simulink model "hw_BuildIn_Gyro"  (R2020b)
settings: Solver=FixedStepAuto  StartTime=0.0  StopTime=inf  RelTol=1e-3  EnableMultiTasking=on
libraries: arduinolib x10, simulink x4
settings Model: SILPILModeSetting=veronly  EnablePacing=on  ExtModeTrigDuration=2  Creator=IDE-Admin  LastModifiedBy=helve
settings OptimizationCC: EnhancedBackFolding=on  PassReuseOutputArgsAs=Individual arguments  ZeroExternalMemoryAtStartup=off  ZeroInternalMemoryAtStartup=off  MaxStackSize=64  OptimizeBlockOrder=speed  DifferentSizesBufferReuse=on  OptimizationCustomize=off  EfficientTunableParamExpr=on
settings DebuggingCC: ParameterTunabilityLossMsg=error
settings HardwareCC: ProdBitPerPointer=32  ProdBitPerSizeT=32  ProdBitPerPtrDiffT=32  ProdLargestAtomicInteger=Long  ProdLargestAtomicFloat=Double  ProdWordSize=32  ProdHWDeviceType=ARM Compatible->ARM Cortex
settings SFSimCC: MATLABDynamicMemAlloc=off
settings RTWCC: Description=Embedded Coder  SystemTargetFile=ert.tlc  HardwareBoard=Arduino Nano 33 IoT  TemplateMakefile=ert_default_tmf  Toolchain=Arduino ARM  BuildConfiguration=Faster Runs
settings CodeAppCC: ForceParamTrailComments=on  IgnoreCustomStorageClasses=off  OperatorAnnotations=on  SimulinkDataObjDesc=on  SFDataObjDesc=on  InsertBlockDesc=on
settings ERTTargetCC: SupportContinuousTime=on  SupportVariableSizeSignals=on  ExtModeTransport=3  ExtModeStaticAllocSize=8192  ExtModeMexFile=ext_xcp  ExtModeIntrfLevel=Level2 - Open

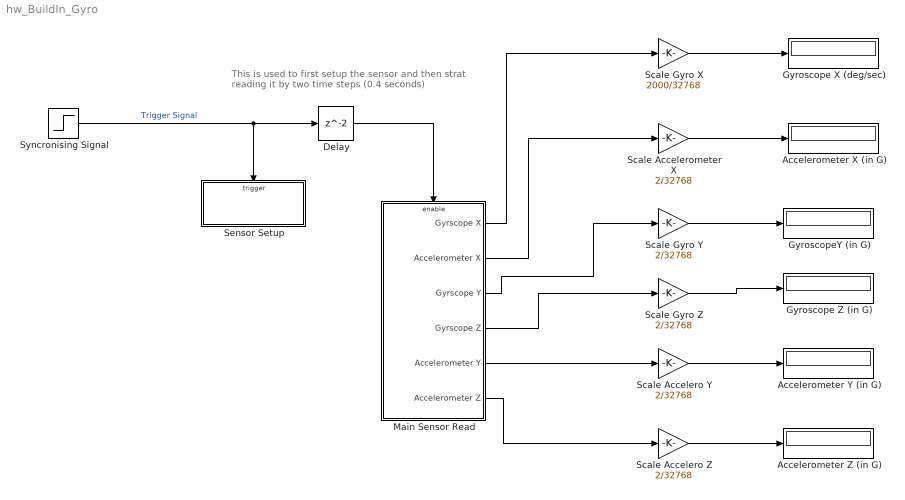
== system hw_BuildIn_Gyro ==
  note: This is used to first setup the sensor and
      | then strat reading it by two time steps (0.4 seconds)
  Accelerometer X (in G) : Display
  Accelerometer Y (in G) : Display
  Accelerometer Z (in G) : Display
  Delay : Delay
  Gyroscope X (deg/sec) : Display
  Gyroscope Z (in G) : Display
  GyroscopeY (in G) : Display
  Main Sensor Read : Subsystem  TreatAsAtomicUnit=on
  Scale Accelero Y : Gain  Gain=2/32768  OutDataTypeStr=single
  Scale Accelero Z : Gain  Gain=2/32768  OutDataTypeStr=single
  Scale Accelerometer X : Gain  Gain=2/32768  OutDataTypeStr=single
  Scale Gyro X : Gain  Gain=2000/32768  OutDataTypeStr=single
  Scale Gyro Y : Gain  Gain=2/32768  OutDataTypeStr=single
  Scale Gyro Z : Gain  Gain=2/32768  OutDataTypeStr=single
  Sensor Setup : Subsystem  TreatAsAtomicUnit=on
  Syncronising Signal : Step
  wires:
  Syncronising Signal/1 -> Sensor Setup/Trigger, Delay/1  "Trigger Signal"
  Delay/1 -> Main Sensor Read/Enable
  Main Sensor Read/1(Gyrscope X) -> Scale Gyro X/1
  Scale Gyro X/1 -> Gyroscope X (deg/sec)/1
  Scale Accelerometer X/1 -> Accelerometer X (in G)/1
  Main Sensor Read/2(Accelerometer X) -> Scale Accelerometer X/1
  Scale Gyro Y/1 -> GyroscopeY (in G)/1
  Main Sensor Read/3(Gyrscope Y) -> Scale Gyro Y/1
  Scale Gyro Z/1 -> Gyroscope Z (in G)/1
  Main Sensor Read/4(Gyrscope Z) -> Scale Gyro Z/1
  Scale Accelero Y/1 -> Accelerometer Y (in G)/1
  Main Sensor Read/5(Accelerometer Y) -> Scale Accelero Y/1
  Scale Accelero Z/1 -> Accelerometer Z (in G)/1
  Main Sensor Read/6(Accelerometer Z) -> Scale Accelero Z/1

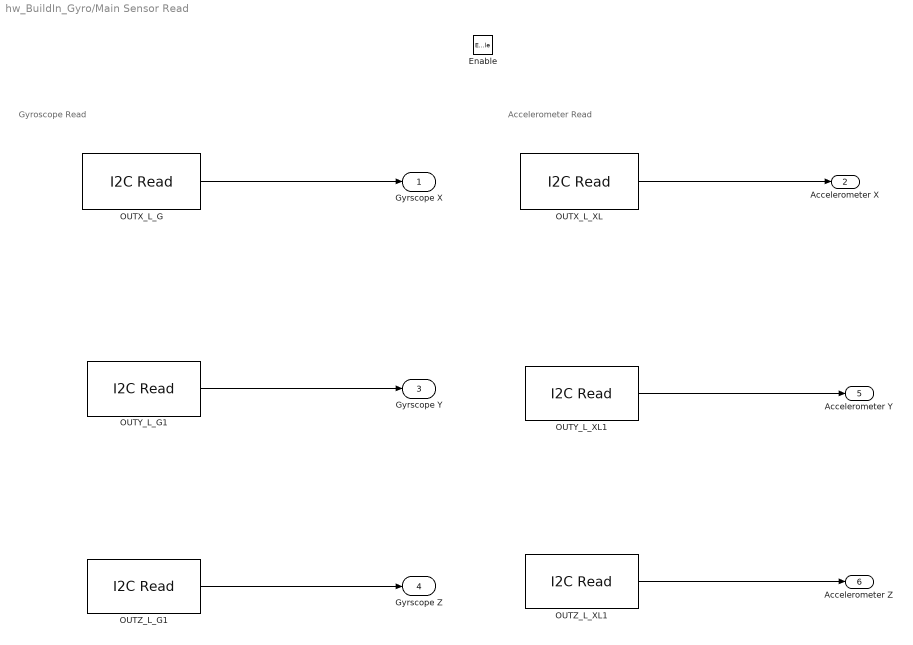
== system hw_BuildIn_Gyro/Main Sensor Read ==
  note: Gyroscope Read
  note: Accelerometer Read
  Enable : EnablePort
  OUTX_L_G : arduinolib/I2C Read  I2CModule=0  Mode=Master  SlaveAddress=0b01101010  SlaveByteOrder=LittleEndian  Direction=Receiver  RegisterAddressMode=on  RegisterAddress=0x22  SlaveDataType=int16  DataLength=1  NoAck=off  RepeatedStart=off  OutputStatus=off  blockPlatform=arduino  SampleTime=-1
      settings: SourceProductBaseCode=ARDUINO
      settings: AttributesFormatString=|
      | %<RegisterAddress>
      | %<SlaveDataType>
  OUTX_L_XL : arduinolib/I2C Read  I2CModule=0  Mode=Master  SlaveAddress=0b01101010  SlaveByteOrder=LittleEndian  Direction=Receiver  RegisterAddressMode=on  RegisterAddress=0x28  SlaveDataType=int16  DataLength=1  NoAck=off  RepeatedStart=off  OutputStatus=off  blockPlatform=arduino  SampleTime=-1
      settings: SourceProductBaseCode=ARDUINO
      settings: AttributesFormatString=|
      | %<RegisterAddress>
      | %<SlaveDataType>
  OUTY_L_G1 : arduinolib/I2C Read  I2CModule=0  Mode=Master  SlaveAddress=0b01101010  SlaveByteOrder=LittleEndian  Direction=Receiver  RegisterAddressMode=on  RegisterAddress=0x24  SlaveDataType=int16  DataLength=1  NoAck=off  RepeatedStart=off  OutputStatus=off  blockPlatform=ARDUINO  SampleTime=-1
      settings: SourceProductBaseCode=ARDUINO
      settings: AttributesFormatString=|
      | %<RegisterAddress>
      | %<SlaveDataType>
  OUTY_L_XL1 : arduinolib/I2C Read  I2CModule=0  Mode=Master  SlaveAddress=0b01101010  SlaveByteOrder=LittleEndian  Direction=Receiver  RegisterAddressMode=on  RegisterAddress=0x2A  SlaveDataType=int16  DataLength=1  NoAck=off  RepeatedStart=off  OutputStatus=off  blockPlatform=ARDUINO  SampleTime=-1
      settings: SourceProductBaseCode=ARDUINO
      settings: AttributesFormatString=|
      | %<RegisterAddress>
      | %<SlaveDataType>
  OUTZ_L_G1 : arduinolib/I2C Read  I2CModule=0  Mode=Master  SlaveAddress=0b01101010  SlaveByteOrder=LittleEndian  Direction=Receiver  RegisterAddressMode=on  RegisterAddress=0x26  SlaveDataType=int16  DataLength=1  NoAck=off  RepeatedStart=off  OutputStatus=off  blockPlatform=ARDUINO  SampleTime=-1
      settings: SourceProductBaseCode=ARDUINO
      settings: AttributesFormatString=|
      | %<RegisterAddress>
      | %<SlaveDataType>
  OUTZ_L_XL1 : arduinolib/I2C Read  I2CModule=0  Mode=Master  SlaveAddress=0b01101010  SlaveByteOrder=LittleEndian  Direction=Receiver  RegisterAddressMode=on  RegisterAddress=0x2C  SlaveDataType=int16  DataLength=1  NoAck=off  RepeatedStart=off  OutputStatus=off  blockPlatform=ARDUINO  SampleTime=-1
      settings: SourceProductBaseCode=ARDUINO
      settings: AttributesFormatString=|
      | %<RegisterAddress>
      | %<SlaveDataType>
  Gyrscope X : Outport  VectorParamsAs1DForOutWhenUnconnected=off
  Accelerometer X : Outport  Port=2  VectorParamsAs1DForOutWhenUnconnected=off
  Gyrscope Y : Outport  Port=3  VectorParamsAs1DForOutWhenUnconnected=off
  Gyrscope Z : Outport  Port=4  VectorParamsAs1DForOutWhenUnconnected=off
  Accelerometer Y : Outport  Port=5  VectorParamsAs1DForOutWhenUnconnected=off
  Accelerometer Z : Outport  Port=6  VectorParamsAs1DForOutWhenUnconnected=off
  wires:
  OUTX_L_G/1 -> Gyrscope X/1
  OUTX_L_XL/1 -> Accelerometer X/1
  OUTY_L_G1/1 -> Gyrscope Y/1
  OUTZ_L_G1/1 -> Gyrscope Z/1
  OUTZ_L_XL1/1 -> Accelerometer Z/1
  OUTY_L_XL1/1 -> Accelerometer Y/1

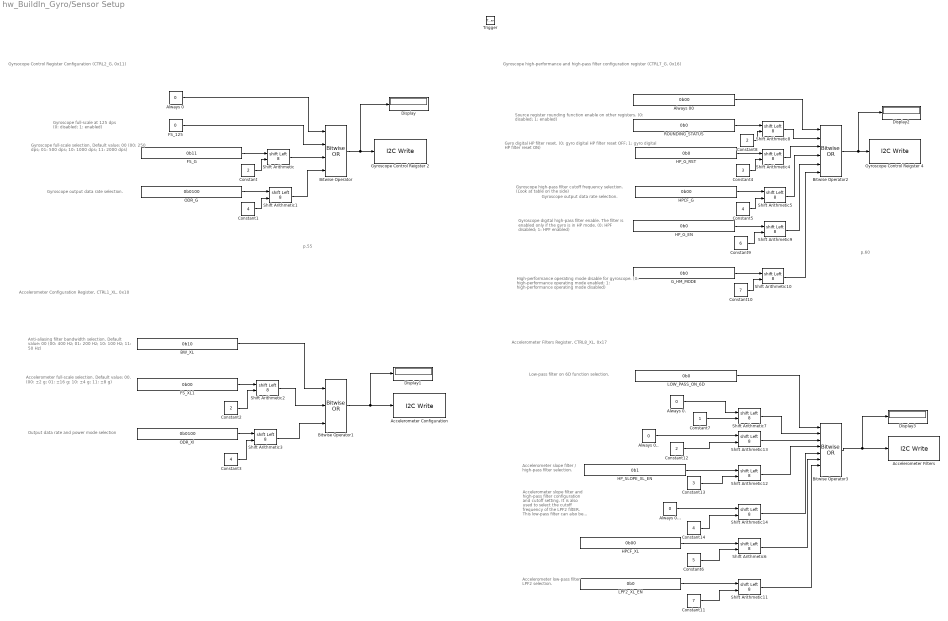
== system hw_BuildIn_Gyro/Sensor Setup ==
  note: Gyroscope high-pass filter cutoff frequency selection.
      | (Look at table on the side)
  note: Gyro digital HP filter reset.
      | (0: gyro digital HP filter reset OFF; 1: gyro digital HP filter reset ON)
  note: p.55
  note: Gyrsocope Control Register Configuration (CTRL2_G, 0x11)
  note: Gyroscope output data rate selection.
  note: Gyroscope full-scale at 125 dps
      | (0: disabled; 1: enabled)
  note: Gyroscope full-scale selection. Default value: 00
      | (00: 250 dps; 01: 500 dps; 10: 1000 dps; 11: 2000 dps)
  note: p.60
  note: Gyroscope high-performance and high-pass filter configuration register (CTRL7_G, 0x16)
  note: Gyroscope output data rate selection.
  note: Source register rounding function enable on other registers.
      | (0: disabled; 1: enabled)
  note: Gyroscope digital high-pass filter enable.
      | The filter is enabled only if the gyro is in HP mode.
      | (0: HPF disabled; 1: HPF enabled)
  note: High-performance operating mode disable for gyroscope.
      | (0: high-performance operating mode enabled;
      | 1: high-performance operating mode disabled)
  note: Accelerometer full-scale selection. Default value: 00. (00: ±2 g; 01: ±16 g; 10: ±4 g; 11: ±8 g)
  note: Output data rate and power mode selection
  note: Accelerometer Configuration Register, CTRL1_XL, 0x10
  note: Anti-aliasing filter bandwidth selection. Default value: 00 (00: 400 Hz; 01: 200 Hz; 10: 100 Hz; 11: 50 Hz)
  note: Low-pass filter on 6D function selection.
  note: Accelerometer Filters Register, CTRL8_XL, 0x17
  note: Accelerometer slope filter and high-pass filter configuration and cutoff setting. It is also used to select the cutoff frequency of the LPF2 filtER. This low-pass filter can also be used in the 6D/4D functionality by setting the LOW_PASS_ON_6D bit of CTRL8_XL (17h) to 1 .
  note: Accelerometer slope filter / high-pass filter selection.
  note: Accelerometer low-pass filter LPF2 selection.
  Trigger : TriggerPort  VariantControl=Variant
  Accelerometer Configuration : arduinolib/I2C Write  Priority=1  I2CModule=0  Mode=Master  SlaveAddress=0b01101010  SlaveByteOrder=BigEndian  Direction=Transmitter  RegisterAddressMode=on  RegisterAddress=0x10  SlaveDataType=uint8  DataLength=1  NoAck=off  RepeatedStart=off  OutputStatus=off  blockPlatform=ARDUINO
      settings: SourceProductBaseCode=ARDUINO
      settings: AttributesFormatString=|
      | Register
      | %<RegisterAddress>
  Accelerometer Filters : arduinolib/I2C Write  Priority=1  I2CModule=0  Mode=Master  SlaveAddress=0b01101010  SlaveByteOrder=BigEndian  Direction=Transmitter  RegisterAddressMode=on  RegisterAddress=0x17  SlaveDataType=uint8  DataLength=1  NoAck=off  RepeatedStart=off  OutputStatus=off  blockPlatform=ARDUINO
      settings: SourceProductBaseCode=ARDUINO
      settings: AttributesFormatString=|
      | Register
      | %<RegisterAddress>
  Always 0 : Constant  Value=0  OutDataTypeStr=uint8  SampleTime=-1
  Always 0. : Constant  Value=0  OutDataTypeStr=uint8  SampleTime=-1
  Always 0.. : Constant  Value=0  OutDataTypeStr=uint8  SampleTime=-1
  Always 0... : Constant  Value=0  OutDataTypeStr=uint8  SampleTime=-1
  Always 00 : Constant  Value=0b00  OutDataTypeStr=uint8  SampleTime=-1
  BW_XL : Constant  Value=0b10  OutDataTypeStr=uint8  SampleTime=-1
  Bitwise Operator : simulink/Logic and Bit Operations/Bitwise Operator  logicop=OR  UseBitMask=off  NumInputPorts=4  BitMask=bin2dec('11011001')  BitMaskRealWorld=Stored Integer
  Bitwise Operator1 : simulink/Logic and Bit Operations/Bitwise Operator  logicop=OR  UseBitMask=off  NumInputPorts=3  BitMask=bin2dec('11011001')  BitMaskRealWorld=Stored Integer
  Bitwise Operator2 : simulink/Logic and Bit Operations/Bitwise Operator  logicop=OR  UseBitMask=off  NumInputPorts=6  BitMask=bin2dec('11011001')  BitMaskRealWorld=Stored Integer
  Bitwise Operator3 : simulink/Logic and Bit Operations/Bitwise Operator  logicop=OR  UseBitMask=off  NumInputPorts=8  BitMask=bin2dec('11011001')  BitMaskRealWorld=Stored Integer
  Constant : Constant  Value=2  OutDataTypeStr=uint8  SampleTime=-1
  Constant1 : Constant  Value=4  OutDataTypeStr=uint16  SampleTime=-1
  Constant10 : Constant  Value=7  OutDataTypeStr=uint8  SampleTime=-1
  Constant11 : Constant  Value=7  OutDataTypeStr=uint16  SampleTime=-1
  Constant12 : Constant  Value=2  OutDataTypeStr=uint16  SampleTime=-1
  Constant13 : Constant  Value=3  OutDataTypeStr=uint16  SampleTime=-1
  Constant14 : Constant  Value=4  OutDataTypeStr=uint16  SampleTime=-1
  Constant2 : Constant  Value=2  OutDataTypeStr=uint16  SampleTime=-1
  Constant3 : Constant  Value=4  OutDataTypeStr=uint16  SampleTime=-1
  Constant4 : Constant  Value=3  OutDataTypeStr=uint8  SampleTime=-1
  Constant5 : Constant  Value=4  OutDataTypeStr=uint8  SampleTime=-1
  Constant6 : Constant  Value=5  OutDataTypeStr=uint16  SampleTime=-1
  Constant7 : Constant  OutDataTypeStr=uint16  SampleTime=-1
  Constant8 : Constant  Value=2  OutDataTypeStr=uint8  SampleTime=-1
  Constant9 : Constant  Value=6  OutDataTypeStr=uint8  SampleTime=-1
  Display{,1..3} (4 alike) : Display
      settings: Format=hex (Stored Integer)
  FS_125 : Constant  Value=0  OutDataTypeStr=uint8  SampleTime=-1
  FS_G : Constant  Value=0b11  OutDataTypeStr=uint8  SampleTime=-1
  FS_XL1 : Constant  Value=0b00  OutDataTypeStr=uint8  SampleTime=-1
  "G_HM_MODE " : Constant  Value=0b0  OutDataTypeStr=uint8  SampleTime=-1
  Gyroscope Control Reigster 2 : arduinolib/I2C Write  I2CModule=0  Mode=Master  SlaveAddress=0b01101010  SlaveByteOrder=BigEndian  Direction=Transmitter  RegisterAddressMode=on  RegisterAddress=0x11  SlaveDataType=uint8  DataLength=1  NoAck=off  RepeatedStart=off  OutputStatus=off  blockPlatform=ARDUINO
      settings: SourceProductBaseCode=ARDUINO
      settings: AttributesFormatString=|
      | Register
      | %<RegisterAddress>
  Gyroscope Control Reigster 4 : arduinolib/I2C Write  I2CModule=0  Mode=Master  SlaveAddress=0b01101010  SlaveByteOrder=BigEndian  Direction=Transmitter  RegisterAddressMode=on  RegisterAddress=0x16  SlaveDataType=uint8  DataLength=1  NoAck=off  RepeatedStart=off  OutputStatus=off  blockPlatform=ARDUINO
      settings: SourceProductBaseCode=ARDUINO
      settings: AttributesFormatString=|
      | Register
      | %<RegisterAddress>
  HPCF_G : Constant  Value=0b00  OutDataTypeStr=uint8  SampleTime=-1
  HPCF_XL : Constant  Value=0b00  OutDataTypeStr=uint8  SampleTime=-1
  HP_G_EN : Constant  Value=0b0  OutDataTypeStr=uint8  SampleTime=-1
  HP_G_RST : Constant  Value=0b0  OutDataTypeStr=uint8  SampleTime=-1
  HP_SLOPE_XL_EN : Constant  Value=0b1  OutDataTypeStr=uint8  SampleTime=-1
  LOW_PASS_ON_6D : Constant  Value=0b0  OutDataTypeStr=uint8  SampleTime=-1
  LPF2_XL_EN : Constant  Value=0b0  OutDataTypeStr=uint8  SampleTime=-1
  "ODR_G " : Constant  Value=0b0100  OutDataTypeStr=uint8  SampleTime=-1
  ODR_Xl : Constant  Value=0b0100  OutDataTypeStr=uint8  SampleTime=-1
  ROUNDING_STATUS : Constant  Value=0b0  OutDataTypeStr=uint8  SampleTime=-1
  Shift Arithmetic{,1..14} (15 alike) : ArithShift  BitShiftNumberSource=Input port  BitShiftNumber=8  BitShiftDirection=Left
      settings: InputPortMap=u0,p1
  wires:
  Constant/1 -> Shift Arithmetic/2
  "ODR_G "/1 -> Shift Arithmetic1/1
  Constant1/1 -> Shift Arithmetic1/2
  FS_G/1 -> Shift Arithmetic/1
  Bitwise Operator/1 -> Display/1, Gyroscope Control Reigster 2/1
  Always 0/1 -> Bitwise Operator/1
  FS_125/1 -> Bitwise Operator/2
  Shift Arithmetic/1 -> Bitwise Operator/3
  Shift Arithmetic1/1 -> Bitwise Operator/4
  Always 00/1 -> Bitwise Operator2/1
  HP_G_RST/1 -> Shift Arithmetic4/1
  Shift Arithmetic4/1 -> Bitwise Operator2/3
  Constant5/1 -> Shift Arithmetic5/2
  HPCF_G/1 -> Shift Arithmetic5/1
  Constant4/1 -> Shift Arithmetic4/2
  Bitwise Operator2/1 -> Display2/1, Gyroscope Control Reigster 4/1
  Shift Arithmetic5/1 -> Bitwise Operator2/4
  ROUNDING_STATUS/1 -> Shift Arithmetic8/1
  Shift Arithmetic8/1 -> Bitwise Operator2/2
  Constant8/1 -> Shift Arithmetic8/2
  HP_G_EN/1 -> Shift Arithmetic9/1
  Constant9/1 -> Shift Arithmetic9/2
  Shift Arithmetic9/1 -> Bitwise Operator2/5
  "G_HM_MODE "/1 -> Shift Arithmetic10/1
  Constant10/1 -> Shift Arithmetic10/2
  Shift Arithmetic10/1 -> Bitwise Operator2/6
  Shift Arithmetic3/1 -> Bitwise Operator1/3
  Bitwise Operator1/1 -> Accelerometer Configuration/1, Display1/1
  Shift Arithmetic2/1 -> Bitwise Operator1/2
  Constant2/1 -> Shift Arithmetic2/2
  BW_XL/1 -> Bitwise Operator1/1
  FS_XL1/1 -> Shift Arithmetic2/1
  ODR_Xl/1 -> Shift Arithmetic3/1
  Constant3/1 -> Shift Arithmetic3/2
  Bitwise Operator3/1 -> Accelerometer Filters/1, Display3/1
  Constant13/1 -> Shift Arithmetic12/2
  Constant14/1 -> Shift Arithmetic14/2
  Constant7/1 -> Shift Arithmetic7/2
  Shift Arithmetic12/1 -> Bitwise Operator3/4
  Constant6/1 -> Shift Arithmetic6/2
  Always 0../1 -> Shift Arithmetic13/1
  HP_SLOPE_XL_EN/1 -> Shift Arithmetic12/1
  Shift Arithmetic14/1 -> Bitwise Operator3/5
  Shift Arithmetic6/1 -> Bitwise Operator3/6
  Shift Arithmetic7/1 -> Bitwise Operator3/2
  LPF2_XL_EN/1 -> Shift Arithmetic11/1
  HPCF_XL/1 -> Shift Arithmetic6/1
  Always 0./1 -> Shift Arithmetic7/1
  Constant11/1 -> Shift Arithmetic11/2
  Shift Arithmetic11/1 -> Bitwise Operator3/7
  Constant12/1 -> Shift Arithmetic13/2
  Always 0.../1 -> Shift Arithmetic14/1
  Shift Arithmetic13/1 -> Bitwise Operator3/3
  LOW_PASS_ON_6D/1 -> Bitwise Operator3/1
